simulink model "Ex22"  (R2019b)
settings: Solver=VariableStepAuto  StartTime=0.0  StopTime=100  RelTol=1e-3
values from neighbouring files (symbols this model uses):
  D = D_v(i)    [Ex_10.m]    (also in Ex_20.m = 3000; Ex_22.m = 0.4; Ex_23.m = 0.1; Ex_29.m = 0.1)
  g = 9.8    [Ex_19.m]    (also in Ex_22.m)
  J = 0.4    [Ex_21.m]    (also in Ex_22.m = 1; Ex_23.m = 1.1; Ex_29.m = 1.1; Untitled2.m = 1)
  K = 1    [Ex_10.m]    (also in Ex_21.m; Ex_22.m; Ex_24.m = 1 / qsi^2; Ex_31.m = 4.26)
  M = 1    [Ex_10.m]    (also in Ex_22.m = 5)
  R = 0.2    [Ex_21.m]    (also in Ex_22.m; Ex_23.m = 1.3; Ex_27.m = 2*qsi * sqrt(L/C); Ex_29.m = 1.3)
settings Model: Creator=andre  LastModifiedBy=andre

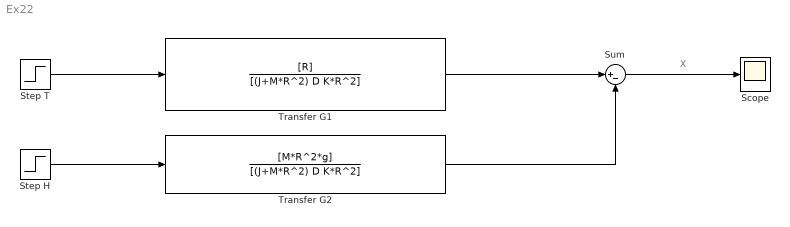
== system Ex22 ==
  note: X
  Scope : Scope
  Step H : Step  Time=0  SampleTime=0
  Step T : Step  Time=0  After=10  SampleTime=0
  Sum : Sum  Inputs=|+-
  Transfer G1 : TransferFcn  Numerator=[R]  Denominator=[(J+M*R^2) D K*R^2]
  Transfer G2 : TransferFcn  Numerator=[M*R^2*g]  Denominator=[(J+M*R^2) D K*R^2]
  wires:
  Transfer G1/1 -> Sum/1
  Transfer G2/1 -> Sum/2
  Sum/1 -> Scope/1
  Step T/1 -> Transfer G1/1
  Step H/1 -> Transfer G2/1
